simulink model "single_reference"  (R2020a)
settings: Solver=VariableStepAuto  StartTime=0.0  StopTime=options.T_train  RelTol=1e-3
settings Model: Creator=kekatos  LastModifiedBy=kekatos

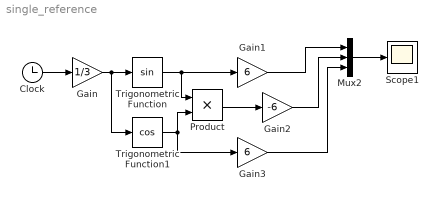
== system single_reference ==
  Clock : Clock
  Gain : Gain  Gain=1/3
  Gain1 : Gain  Gain=6
  Gain2 : Gain  Gain=-6
  Gain3 : Gain  Gain=6
  Mux2 : Mux  Inputs=3
  Product : Product
  Scope1 : Scope
  Trigonometric Function : Trigonometry
  Trigonometric Function1 : Trigonometry  Operator=cos
  wires:
  Clock/1 -> Gain/1
  Mux2/1 -> Scope1/1
  Gain2/1 -> Mux2/2
  Trigonometric Function/1 -> Product/1, Gain1/1
  Trigonometric Function1/1 -> Gain3/1, Product/2
  Gain3/1 -> Mux2/3
  Gain/1 -> Trigonometric Function1/1, Trigonometric Function/1
  Gain1/1 -> Mux2/1
  Product/1 -> Gain2/1
